simulink model "DroneSystem"  (R2016a)
settings: Solver=FixedStepDiscrete  StartTime=0.0  StopTime=10  FixedStep=0.001  RelTol=1e-3
libraries: simulink x1
settings Model: Creator=SEP25  LastModifiedBy=SEP25

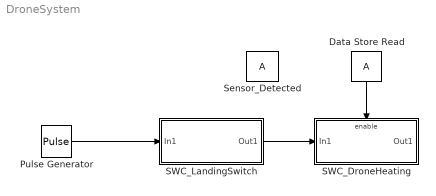
== system DroneSystem ==
  Data Store Read : DataStoreRead
  Pulse Generator : DiscretePulseGenerator  PulseType=Time based  Period=1  PulseWidth=50
  SWC_DroneHeating : Subsystem  TreatAsAtomicUnit=on
  SWC_LandingSwitch : Subsystem
  Sensor_Detected : DataStoreMemory  ReadBeforeWriteMsg=warning  WriteAfterWriteMsg=warning  WriteAfterReadMsg=warning  ShowAdditionalParam=off
  wires:
  Pulse Generator/1 -> SWC_LandingSwitch/1(In1)
  Data Store Read/1 -> SWC_DroneHeating/Enable
  SWC_LandingSwitch/1(Out1) -> SWC_DroneHeating/1(In1)

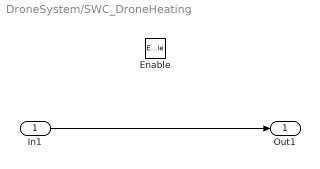
== system DroneSystem/SWC_DroneHeating ==
  In1 : Inport
  Enable : EnablePort
  Out1 : Outport
  wires:
  In1/1 -> Out1/1

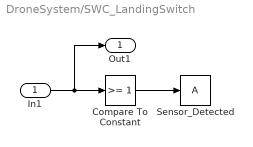
== system DroneSystem/SWC_LandingSwitch ==
  In1 : Inport
  Compare To Constant : simulink/Logic and Bit Operations/Compare To Constant  relop=>=  const=1  OutDataTypeStr=boolean
  Sensor_Detected : DataStoreWrite
  Out1 : Outport
  wires:
  In1/1 -> Out1/1, Compare To Constant/1
  Compare To Constant/1 -> Sensor_Detected/1
